simulink model "Controlador_ADRC"  (R2025b)
settings: Solver=VariableStepAuto  StartTime=0.0  StopTime=10.0  RelTol=1e-3
undefined symbols (not defined in the file or in its folder): ctrller, scenario
settings Model: Creator=USUARIO  LastModifiedBy=USUARIO

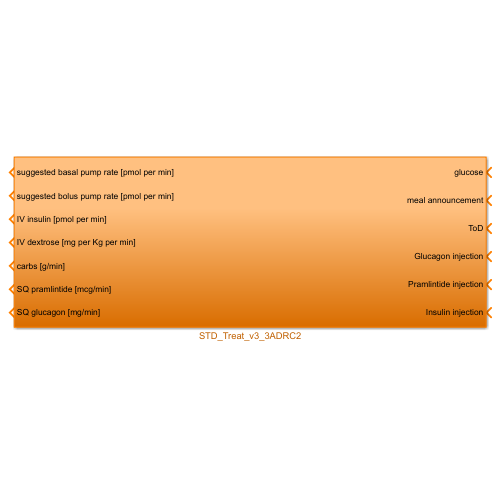
[thumbnail: Simulink's stored preview of the top-level diagram]
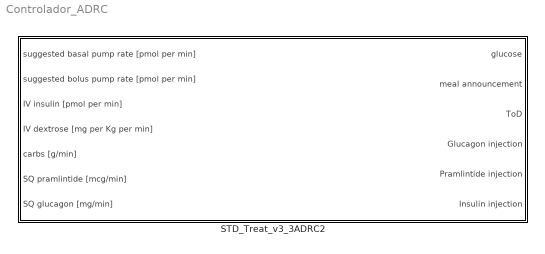
== system Controlador_ADRC ==
  STD_Treat_v3_3ADRC2 : Subsystem

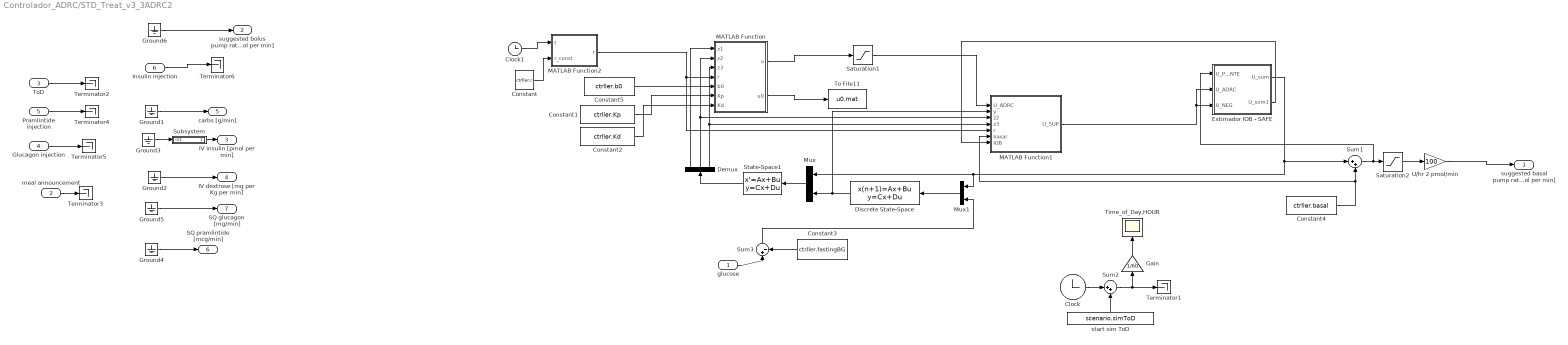
== system Controlador_ADRC/STD_Treat_v3_3ADRC2 ==
  glucose : Inport
  meal announcement : Inport  Port=2
  ToD : Inport  Port=3
  Glucagon injection : Inport  Port=4
  Pramlintide injection : Inport  Port=5
  Insulin injection : Inport  Port=6
  Clock : Clock
  Clock1 : Clock
  Constant : Constant  Value=ctrller.r
  Constant1 : Constant  Value=ctrller.Kp
  Constant2 : Constant  Value=ctrller.Kd
  Constant3 : Constant  Value=ctrller.fastingBG
  Constant4 : Constant  Value=ctrller.basal
  Constant5 : Constant  Value=ctrller.b0
  Demux : Demux  Outputs=3
  Discrete State-Space : DiscreteStateSpace  A=ctrller.KF.Aobs  B=ctrller.KF.Bobs  C=ctrller.KF.Cobs  D=ctrller.KF.Dobs  InitialCondition=ctrller.KF.x0  SampleTime=ctrller.KF.Ts
  Estimador IOB - SAFE : Subsystem
  Gain : Gain  Gain=1/60
  Ground{1..6} (6 alike) : Ground
  MATLAB Function : MATLAB Function  TreatAsAtomicUnit=on
  MATLAB Function1 : MATLAB Function  TreatAsAtomicUnit=on
  MATLAB Function2 : MATLAB Function  TreatAsAtomicUnit=on
  Mux : Mux  Inputs=2
  Mux1 : Mux  Inputs=2
  Saturation1 : Saturate  UpperLimit=ctrller.lim1  LowerLimit=ctrller.lim2
  Saturation2 : Saturate  UpperLimit=8  LowerLimit=0
  State-Space1 : StateSpace  A=ctrller.A_obs  B=ctrller.B_obs  C=ctrller.C_obs  D=ctrller.D_obs  InitialCondition=[0;0;0]
  Subsystem : Subsystem
  Sum1 : Sum  Inputs=|++
  Sum2 : Sum  Inputs=|++
  Sum3 : Sum  Inputs=|+-
  Terminator{1..6} (6 alike) : Terminator
  Time_of_Day,HOUR : Scope
      settings: ActiveDisplayYMinimum=0  ActiveDisplayYMaximum=60000  DataLoggingVariableName=ScopeData22
  To File11 : ToFile  Filename=u0.mat  MatrixName=u0  SaveFormat=Timeseries
  U/hr 2 pmol/min : Gain  Gain=100
  start sim ToD : Constant  Value=scenario.simToD
  suggested basal pump rate [pmol per min] : Outport
  suggested bolus pump rate [pmol per min] : Outport  Port=2
  IV insulin [pmol per min] : Outport  Port=3
  IV dextrose [mg per Kg per min] : Outport  Port=4
  carbs [g/min] : Outport  Port=5
  SQ pramlintide [mcg/min] : Outport  Port=6
  SQ glucagon [mg/min] : Outport  Port=7
  wires:
  Mux1/1 -> Discrete State-Space/1
  Estimador IOB - SAFE/1(U_sum) -> Mux/1, Mux1/1, Sum1/1
  Mux/1 -> State-Space1/1
  Discrete State-Space/1 -> Mux/2, MATLAB Function1/2(y)
  Estimador IOB - SAFE/2(U_sum1) -> MATLAB Function1/7(IOB)
  Sum3/1 -> Mux1/2
  meal announcement/1 -> Terminator3/1
  MATLAB Function/2(u0) -> To File11/1
  Saturation2/1 -> U/hr 2 pmol/min/1
  MATLAB Function/1(u) -> Saturation1/1
  Constant/1 -> MATLAB Function2/2(r_const)
  Demux/3 -> MATLAB Function1/4(z3), MATLAB Function/3(z3)
  glucose/1 -> Sum3/1
  Sum1/1 -> Estimador IOB - SAFE/1(U_PACIENTE), Saturation2/1
  Clock1/1 -> MATLAB Function2/1(t)
  MATLAB Function1/1(U_SUP) -> Estimador IOB - SAFE/3(U_NEG), Estimador IOB - SAFE/2(U_ADRC)
  Constant4/1 -> MATLAB Function1/6(basal), Sum1/2
  Constant3/1 -> Sum3/2
  Saturation1/1 -> MATLAB Function1/1(U_ADRC)
  MATLAB Function2/1(r) -> MATLAB Function/4(r), MATLAB Function1/5(r)
  Demux/2 -> MATLAB Function1/3(z2), MATLAB Function/2(z2)
  Constant2/1 -> MATLAB Function/7(Kd)
  Constant1/1 -> MATLAB Function/6(Kp)
  Demux/1 -> MATLAB Function/1(z1)
  State-Space1/1 -> Demux/1
  Subsystem/1(IV insulin [pmol per min]) -> IV insulin [pmol per min]/1
  Ground3/1 -> Subsystem/1(In1)
  Constant5/1 -> MATLAB Function/5(b0)
  Insulin injection/1 -> Terminator6/1
  Ground1/1 -> carbs [g/min]/1
  Glucagon injection/1 -> Terminator5/1
  Ground2/1 -> IV dextrose [mg per Kg per min]/1
  Pramlintide injection/1 -> Terminator4/1
  Ground4/1 -> SQ pramlintide [mcg/min]/1
  Ground5/1 -> SQ glucagon [mg/min]/1
  Gain/1 -> Time_of_Day,HOUR/1
  start sim ToD/1 -> Sum2/2
  Sum2/1 -> Gain/1, Terminator1/1
  Clock/1 -> Sum2/1
  ToD/1 -> Terminator2/1
  U/hr 2 pmol/min/1 -> suggested basal pump rate [pmol per min]/1
  Ground6/1 -> suggested bolus pump rate [pmol per min]/1

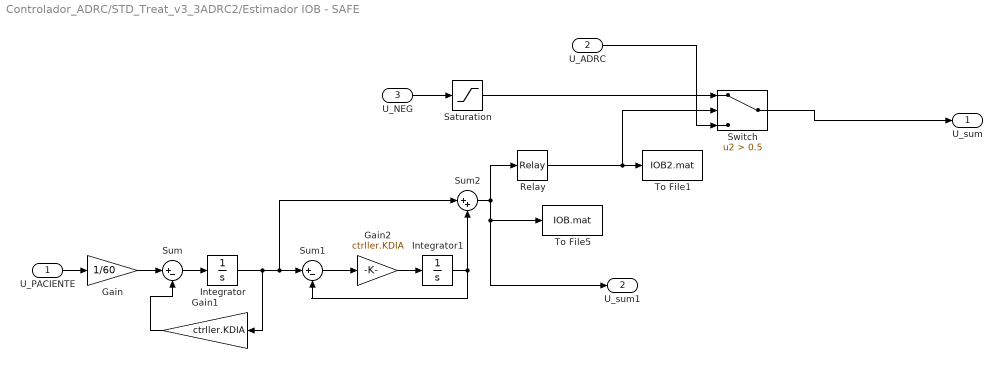
== system Controlador_ADRC/STD_Treat_v3_3ADRC2/Estimador IOB - SAFE ==
  U_PACIENTE : Inport
  U_ADRC : Inport  Port=2
  U_NEG : Inport  Port=3
  Gain : Gain  Gain=1/60
  Gain1 : Gain  Gain=ctrller.KDIA
  Gain2 : Gain  Gain=ctrller.KDIA
  Integrator : Integrator
  Integrator1 : Integrator
  Relay : Relay  OnSwitchValue=ctrller.sw  OffSwitchValue=ctrller.swneg
  Saturation : Saturate  UpperLimit=0  LowerLimit=-1000  ZeroCross=off
  Sum : Sum  Inputs=|+-
  Sum1 : Sum  Inputs=|+-
  Sum2 : Sum  Inputs=|++
  Switch : Switch  Criteria=u2 > Threshold  Threshold=0.5  SaturateOnIntegerOverflow=off  InputSameDT=off
  To File1 : ToFile  Filename=IOB2.mat  MatrixName=IOB2  SaveFormat=Timeseries
  To File5 : ToFile  Filename=IOB.mat  MatrixName=IOB  SaveFormat=Timeseries
  U_sum : Outport
  U_sum1 : Outport  Port=2
  wires:
  U_ADRC/1 -> Switch/3
  Saturation/1 -> Switch/1
  Switch/1 -> U_sum/1
  U_NEG/1 -> Saturation/1
  Relay/1 -> Switch/2, To File1/1
  Sum2/1 -> To File5/1, U_sum1/1, Relay/1
  Integrator1/1 -> Sum1/2, Sum2/2
  Gain2/1 -> Integrator1/1
  Sum1/1 -> Gain2/1
  Integrator/1 -> Gain1/1, Sum1/1, Sum2/1
  Gain1/1 -> Sum/2
  Sum/1 -> Integrator/1
  Gain/1 -> Sum/1
  U_PACIENTE/1 -> Gain/1

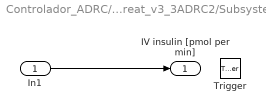
== system Controlador_ADRC/STD_Treat_v3_3ADRC2/Subsystem ==
  In1 : Inport
  Trigger : TriggerPort  VariantControl=(inherit)  PortDimensions=1
  IV insulin [pmol per min] : Outport
  wires:
  In1/1 -> IV insulin [pmol per min]/1

== matlab function Controlador_ADRC/STD_Treat_v3_3ADRC2/MATLAB Function ==
  data: z1 input; z2 input; z3 input; r input; b0 input; u output; Kp input; Kd input; u0 output
function [u,u0] = fcn(z1, z2, z3, r, b0, Kp, Kd)


%% LEY DE CONTROL ORIGINAL
e  = r - z1;
de = -z2;

u01 = Kp*e + Kd*de;
u0  = u01 - z3;
u   = (u01 - z3)/b0;

%% SUMA DEL ANUNCIO DE COMIDA


end

== matlab function Controlador_ADRC/STD_Treat_v3_3ADRC2/MATLAB Function1 ==
  data: U_ADRC input; U_SUP output; y input; z2 input; z3 input; r input; basal input; IOB input
function U_SUP = supervisor_ruido(U_ADRC, y, z2, z3, r, basal, IOB)

%% =========================================================
% SUPERVISOR ADRC + IOB
%
% Objetivo:
% - Mantener la lógica original
% - Evitar acumulación excesiva de insulina
% - Reducir correcciones cuando el IOB ya es alto
%% =========================================================

%% Parámetros originales
deadband = 15;

G_low  = -45;
G_high = 20;

z3_noise = 0.08;
z3_meal  = 0.10;

z2_down1 = -0.25;
z2_down2 = -0.60;

%% =========================================================
% Umbrales nuevos de IOB
%% =========================================================

IOB_soft = 3.5;   % empezar a reducir
IOB_med  = 4.5;   % reducción más fuerte
IOB_high = 5.2;   % limitar agresivamente

%% Salida inicial
U_SUP = U_ADRC;

%% =========================================================
% 1. Seguridad por glucosa baja
%% =========================================================

if y < G_low
    U_SUP = -0.95*basal;
    return
end

%% =========================================================
% 2. Limitación progresiva por IOB
%
% SOLO sobre acción positiva.
%
% No anulamos directamente al ADRC.
%% =========================================================

if U_SUP > 0

    if IOB >= IOB_high

        % Mucha insulina activa:
        % dejar solo una pequeña parte de la corrección
        U_SUP = 0.20*U_SUP;

    elseif IOB >= IOB_med

        % IOB alto
        U_SUP = 0.45*U_SUP;

    elseif IOB >= IOB_soft

        % IOB moderado
        U_SUP = 0.70*U_SUP;

    end

end

%% =========================================================
% 3. Perturbación clara por z3
%
% IMPORTANTE:
% Ya NO hacemos:
%
%   U_SUP = U_ADRC;
%
% porque eso ignoraría la limitación por IOB.
%% =========================================================

if z3 > z3_meal

    % La perturbación existe, pero respetamos la
    % limitación que ya aplicamos según IOB.

    return
end

%% =========================================================
% 4. Cerca de referencia y sin perturbación clara
%% =========================================================

if abs(y-r) < deadband && abs(z3) < z3_noise

    if abs(U_ADRC) < 0.8
        U_SUP = 0;
    end

end

%% =========================================================
% 5. Si la glucosa baja moderadamente
%% =========================================================

if z2 < z2_down1 && U_SUP > 0
    U_SUP = 0.75*U_SUP;
end

%% =========================================================
% 6. Si baja fuerte y ya está baja
%% =========================================================

if z2 < z2_down2 && y < -25

    U_SUP = -0.95*basal;
    return

end

%% =========================================================
% 7. Glucosa alta
%
% Antes hacíamos:
% U_SUP = U_ADRC
%
% Eso volvería a eliminar la protección de IOB.
%
% Ahora simplemente dejamos el valor ya limitado.
%% =========================================================

if y > G_high
    return
end

end

== matlab function Controlador_ADRC/STD_Treat_v3_3ADRC2/MATLAB Function2 ==
  data: t input; r output; r_const input
function r = referencia_horaria(t, r_const)

% t en minutos
% r_const viene de un bloque Constant

if t < 240
    r = 0;          % al inicio apunta a 122 mg/dL

elseif t < 360
    r = r_const*(t-240)/(360-240);  % transición suave

else
    r = r_const;    % referencia final
end

end
